simulink model "MISSILE_2angle"  (R2024b)
settings: Solver=ode4  StartTime=0.0  StopTime=100  FixedStep=0.01  RelTol=1e-3
values from neighbouring files (symbols this model uses):
  Ka = 4.5    [INITIAL_2angle.m]
  Kdc = 1.1    [INITIAL_2angle.m]
  Ki = 14.3    [INITIAL_2angle.m]
  Kr = -0.37    [INITIAL_2angle.m]
  L_M0 = 70*d2r    (= 1.2217304764)    [INITIAL_2angle.m]
  L_T0 = -2.5*d2r    (= -0.0436332312999)    [INITIAL_2angle.m]
  P_M0 = 50*d2r    (= 0.872664625997)    [INITIAL_2angle.m]
  P_T0 = 30*d2r    (= 0.523598775598)    [INITIAL_2angle.m]
  V_T = 600    [INITIAL_2angle.m]
  X_M0 = 0    [INITIAL_2angle.m]
  X_T0 = 0    [INITIAL_2angle.m]
  Y_T0 = 0    [INITIAL_2angle.m]
  Z_M0 = 0    [INITIAL_2angle.m]
  Z_T0 = 20000    [INITIAL_2angle.m]
libraries: simulink x1
settings Model: Creator=Administrator  LastModifiedBy=Administrator

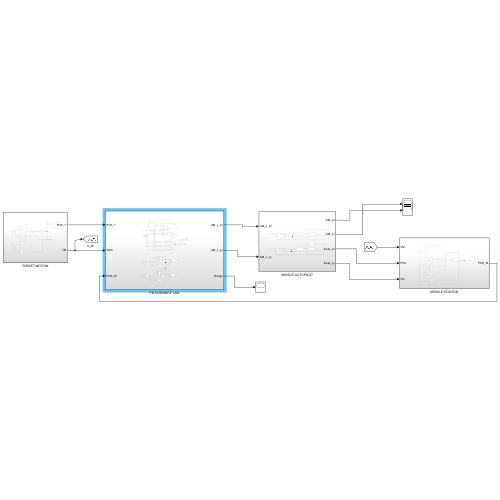
[thumbnail: Simulink's stored preview of the top-level diagram]
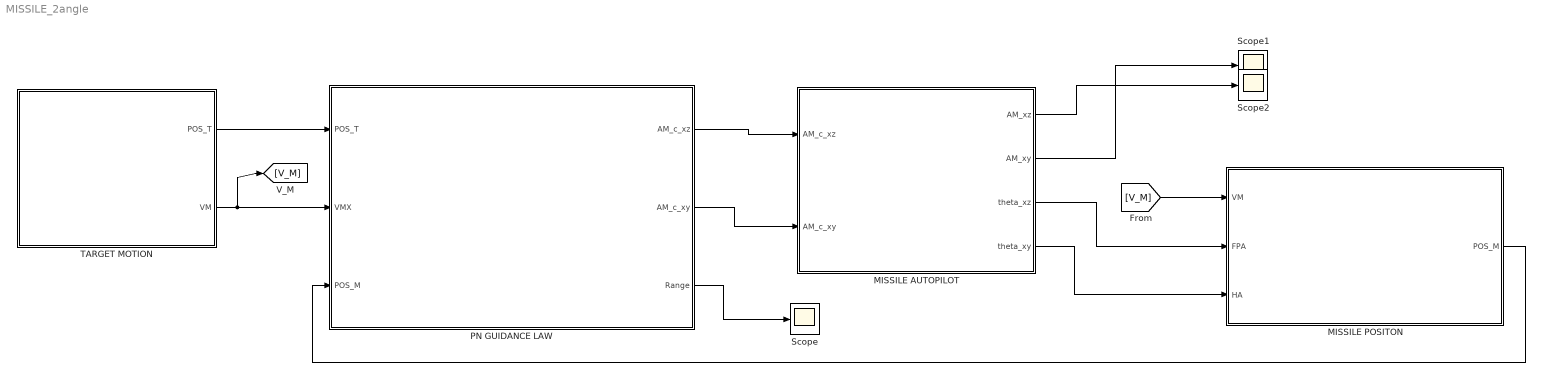
== system MISSILE_2angle ==
  MISSILE AUTOPILOT : Subsystem
  MISSILE POSITON : Subsystem
  PN GUIDANCE LAW : Subsystem
  Scope : Scope
  Scope1 : Scope
  Scope2 : Scope
  TARGET MOTION : Subsystem
  wires:
  TARGET MOTION/1(POS_T) -> PN GUIDANCE LAW/1(POS_T)
  TARGET MOTION/2(VM) -> [V_M], PN GUIDANCE LAW/2(VMX)
  [V_M] -> MISSILE POSITON/1(VM)
  MISSILE POSITON/1(POS_M) -> PN GUIDANCE LAW/3(POS_M)
  PN GUIDANCE LAW/1(AM_c_xz) -> MISSILE AUTOPILOT/1(AM_c_xz)
  MISSILE AUTOPILOT/1(AM_xz) -> Scope2/1
  MISSILE AUTOPILOT/3(theta_xz) -> MISSILE POSITON/2(FPA)
  PN GUIDANCE LAW/3(Range) -> Scope/1
  PN GUIDANCE LAW/2(AM_c_xy) -> MISSILE AUTOPILOT/2(AM_c_xy)
  MISSILE AUTOPILOT/2(AM_xy) -> Scope1/1
  MISSILE AUTOPILOT/4(theta_xy) -> MISSILE POSITON/3(HA)

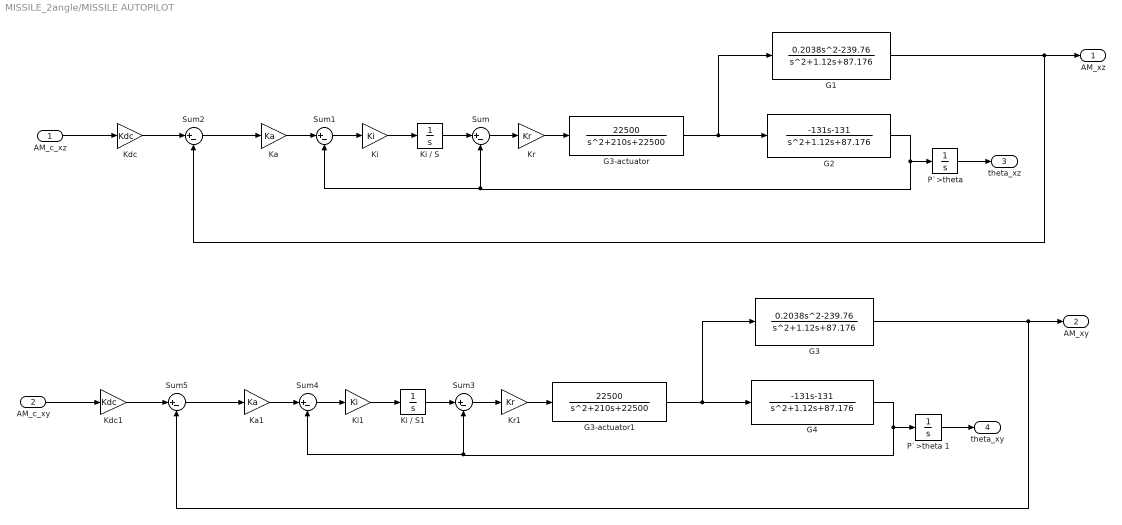
== system MISSILE_2angle/MISSILE AUTOPILOT ==
  AM_c_xz : Inport
  AM_c_xy : Inport  Port=2
  G1 : TransferFcn  Numerator=[0.2038 0 -239.76]  Denominator=[1 1.12 87.176]
  G2 : TransferFcn  Numerator=[-131 -131]  Denominator=[1 1.12 87.176]
  G3 : TransferFcn  Numerator=[0.2038 0 -239.76]  Denominator=[1 1.12 87.176]
  G3-actuator : TransferFcn  Numerator=[22500]  Denominator=[1 210 22500]
  G3-actuator1 : TransferFcn  Numerator=[22500]  Denominator=[1 210 22500]
  G4 : TransferFcn  Numerator=[-131 -131]  Denominator=[1 1.12 87.176]
  Ka : Gain  Gain=Ka
  Ka1 : Gain  Gain=Ka
  Kdc : Gain  Gain=Kdc
  Kdc1 : Gain  Gain=Kdc
  Ki : Gain  Gain=Ki
  Ki / S : Integrator
  Ki / S1 : Integrator
  Ki1 : Gain  Gain=Ki
  Kr : Gain  Gain=Kr
  Kr1 : Gain  Gain=Kr
  "P`>theta " : Integrator  InitialCondition=L_M0
  P`>theta 1 : Integrator  InitialCondition=P_M0
  Sum{,1..5} (6 alike) : Sum  Inputs=|+-
  AM_xz : Outport
  AM_xy : Outport  Port=2
  theta_xz : Outport  Port=3
  theta_xy : Outport  Port=4
  wires:
  Ki / S/1 -> Sum/1
  G1/1 -> AM_xz/1, Sum2/2
  Kr/1 -> G3-actuator/1
  "P`>theta "/1 -> theta_xz/1
  Ka/1 -> Sum1/1
  G3-actuator/1 -> G1/1, G2/1
  Sum1/1 -> Ki/1
  G2/1 -> "P`>theta "/1, Sum1/2, Sum/2
  Kdc/1 -> Sum2/1
  Ki/1 -> Ki / S/1
  Sum/1 -> Kr/1
  Sum2/1 -> Ka/1
  AM_c_xz/1 -> Kdc/1
  P`>theta 1/1 -> theta_xy/1
  Sum3/1 -> Kr1/1
  G4/1 -> P`>theta 1/1, Sum4/2, Sum3/2
  G3-actuator1/1 -> G3/1, G4/1
  AM_c_xy/1 -> Kdc1/1
  Kr1/1 -> G3-actuator1/1
  Ki1/1 -> Ki / S1/1
  G3/1 -> AM_xy/1, Sum5/2
  Ka1/1 -> Sum4/1
  Kdc1/1 -> Sum5/1
  Ki / S1/1 -> Sum3/1
  Sum4/1 -> Ki1/1
  Sum5/1 -> Ka1/1

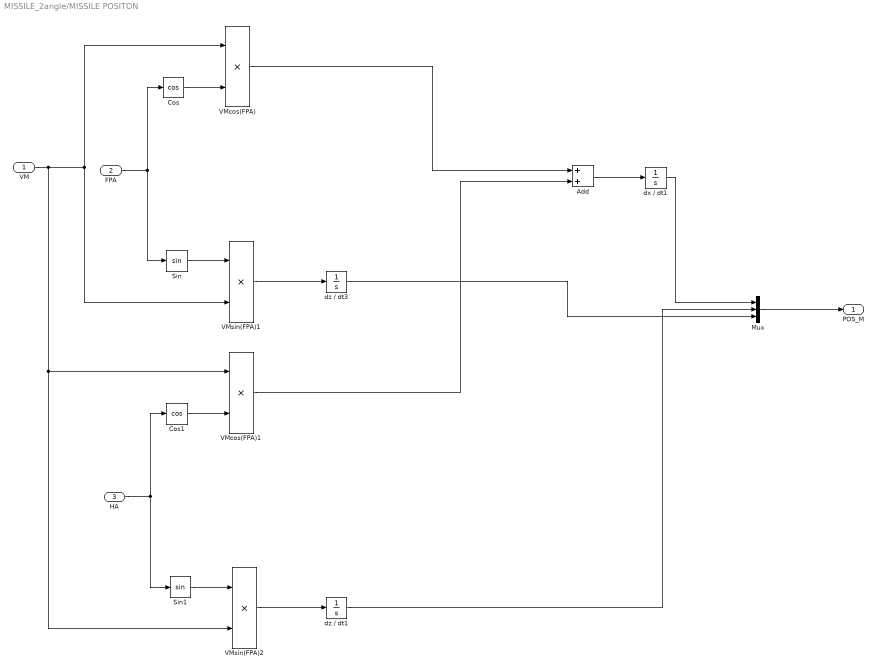
== system MISSILE_2angle/MISSILE POSITON ==
  VM : Inport
  FPA : Inport  Port=2
  HA : Inport  Port=3
  Add : Sum
  Cos : Trigonometry  Operator=cos
  Cos1 : Trigonometry  Operator=cos
  Mux : Mux  Inputs=3
  Sin : Trigonometry
  Sin1 : Trigonometry
  VMcos(FPA) : Product
  VMcos(FPA)1 : Product
  VMsin(FPA)1 : Product
  VMsin(FPA)2 : Product
  dx / dt1 : Integrator  InitialCondition=X_M0
  dz / dt1 : Integrator  InitialCondition=Z_M0
  dz / dt3 : Integrator  InitialCondition=Z_M0
  POS_M : Outport
  wires:
  Sin/1 -> VMsin(FPA)1/1
  Mux/1 -> POS_M/1
  Cos/1 -> VMcos(FPA)/2
  VM/1 -> VMsin(FPA)2/2, VMcos(FPA)1/1, VMsin(FPA)1/2, VMcos(FPA)/1
  FPA/1 -> Sin/1, Cos/1
  Sin1/1 -> VMsin(FPA)2/1
  Cos1/1 -> VMcos(FPA)1/2
  HA/1 -> Sin1/1, Cos1/1
  VMsin(FPA)1/1 -> dz / dt3/1
  VMsin(FPA)2/1 -> dz / dt1/1
  VMcos(FPA)/1 -> Add/1
  Add/1 -> dx / dt1/1
  VMcos(FPA)1/1 -> Add/2
  dz / dt3/1 -> Mux/3
  dz / dt1/1 -> Mux/2
  dx / dt1/1 -> Mux/1

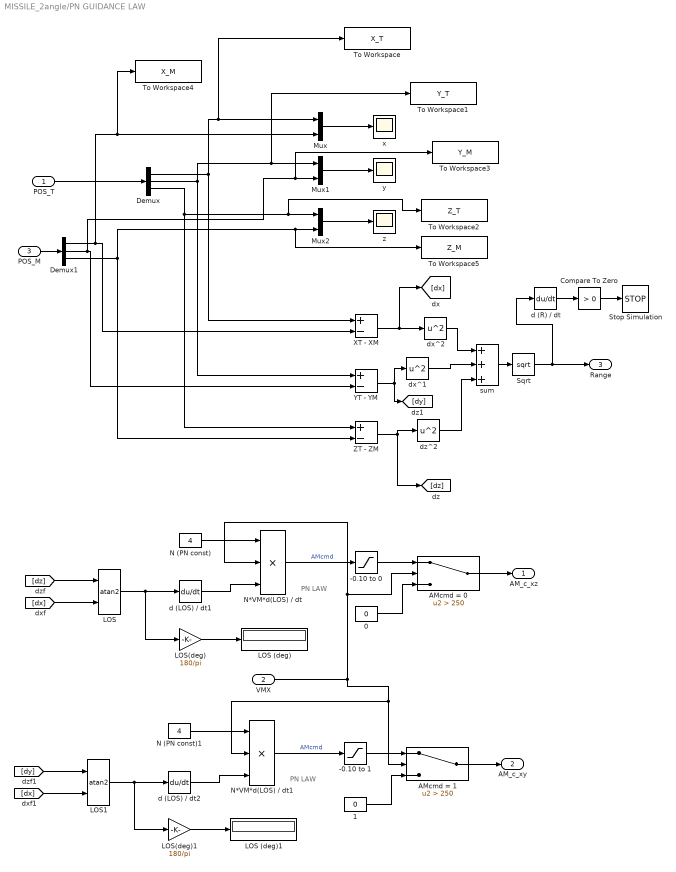
== system MISSILE_2angle/PN GUIDANCE LAW ==
  note: PN LAW
  note: PN LAW
  POS_T : Inport
  VMX : Inport  Port=2
  POS_M : Inport  Port=3
  -0.10 to 0 : Saturate  UpperLimit=1  LowerLimit=-0.1
  -0.10 to 1 : Saturate  UpperLimit=1
  0 : Constant  Value=0
  1 : Constant  Value=0
  AMcmd = 0 : Switch  Criteria=u2 > Threshold  Threshold=250  SaturateOnIntegerOverflow=off  InputSameDT=off
  AMcmd = 1 : Switch  Criteria=u2 > Threshold  Threshold=250  SaturateOnIntegerOverflow=off  InputSameDT=off
  Compare To Zero : simulink/Logic and Bit Operations/Compare To Zero  relop=>  OutDataTypeStr=boolean
  Demux : Demux  Outputs=3
  Demux1 : Demux  Outputs=3
  LOS : Trigonometry  Operator=atan2
  LOS (deg) : Display
  LOS (deg)1 : Display
  LOS(deg) : Gain  Gain=180/pi
  LOS(deg)1 : Gain  Gain=180/pi
  LOS1 : Trigonometry  Operator=atan2
  Mux : Mux  Inputs=2
  Mux1 : Mux  Inputs=2
  Mux2 : Mux  Inputs=2
  N (PN const) : Constant  Value=4
  N (PN const)1 : Constant  Value=4
  N*VM*d(LOS) / dt : Product  Inputs=3
  N*VM*d(LOS) / dt1 : Product  Inputs=3
  Sqrt : Sqrt
  Stop Simulation : Stop
  To Workspace : ToWorkspace  VariableName=X_T  SaveFormat=Timeseries  SampleTime=-1
  To Workspace1 : ToWorkspace  VariableName=Y_T  SaveFormat=Timeseries  SampleTime=-1
  To Workspace2 : ToWorkspace  VariableName=Z_T  SaveFormat=Timeseries  SampleTime=-1
  To Workspace3 : ToWorkspace  VariableName=Y_M  SaveFormat=Timeseries  SampleTime=-1
  To Workspace4 : ToWorkspace  VariableName=X_M  SaveFormat=Timeseries  SampleTime=-1
  To Workspace5 : ToWorkspace  VariableName=Z_M  SaveFormat=Timeseries  SampleTime=-1
  XT - XM : Sum  Inputs=+-
  YT - YM : Sum  Inputs=+-
  ZT - ZM : Sum  Inputs=+-
  d (LOS) / dt1 : Derivative
  d (LOS) / dt2 : Derivative
  d (R) / dt : Derivative
  dx^1 : Math  Operator=square
  dx^2 : Math  Operator=square
  dz^2 : Math  Operator=square
  sum : Sum  Inputs=+++
  x : Scope
  y : Scope
  z : Scope
  AM_c_xz : Outport
  AM_c_xy : Outport  Port=2
  Range : Outport  Port=3
  wires:
  POS_T/1 -> Demux/1
  d (R) / dt/1 -> Compare To Zero/1
  0/1 -> AMcmd = 0/3
  ZT - ZM/1 -> [dz], dz^2/1
  N*VM*d(LOS) / dt/1 -> -0.10 to 0/1  "AMcmd"
  -0.10 to 0/1 -> AMcmd = 0/1
  XT - XM/1 -> [dx], dx^2/1
  LOS/1 -> LOS(deg)/1, d (LOS) / dt1/1
  AMcmd = 0/1 -> AM_c_xz/1
  N (PN const)/1 -> N*VM*d(LOS) / dt/1
  [dx] -> LOS/2
  d (LOS) / dt1/1 -> N*VM*d(LOS) / dt/3
  dx^2/1 -> sum/1
  Compare To Zero/1 -> Stop Simulation/1
  [dz] -> LOS/1
  POS_M/1 -> Demux1/1
  LOS(deg)/1 -> LOS (deg)/1
  Mux1/1 -> y/1
  Mux/1 -> x/1
  dz^2/1 -> sum/3
  Demux/1 -> XT - XM/1, To Workspace/1, Mux/1
  Demux/2 -> To Workspace1/1, Mux1/1, YT - YM/1
  Demux/3 -> To Workspace2/1, Mux2/1, ZT - ZM/1
  Demux1/1 -> Mux/2, To Workspace4/1, XT - XM/2
  Demux1/2 -> To Workspace3/1, Mux1/2, YT - YM/2
  Demux1/3 -> ZT - ZM/2, To Workspace5/1, Mux2/2
  Mux2/1 -> z/1
  YT - YM/1 -> [dy], dx^1/1
  dx^1/1 -> sum/2
  AMcmd = 1/1 -> AM_c_xy/1
  LOS(deg)1/1 -> LOS (deg)1/1
  -0.10 to 1/1 -> AMcmd = 1/1
  N (PN const)1/1 -> N*VM*d(LOS) / dt1/1
  1/1 -> AMcmd = 1/3
  LOS1/1 -> LOS(deg)1/1, d (LOS) / dt2/1
  [dy] -> LOS1/1
  d (LOS) / dt2/1 -> N*VM*d(LOS) / dt1/3
  [dx] -> LOS1/2
  N*VM*d(LOS) / dt1/1 -> -0.10 to 1/1  "AMcmd"
  VMX/1 -> N*VM*d(LOS) / dt/2, AMcmd = 0/2, N*VM*d(LOS) / dt1/2, AMcmd = 1/2
  sum/1 -> Sqrt/1
  Sqrt/1 -> Range/1, d (R) / dt/1

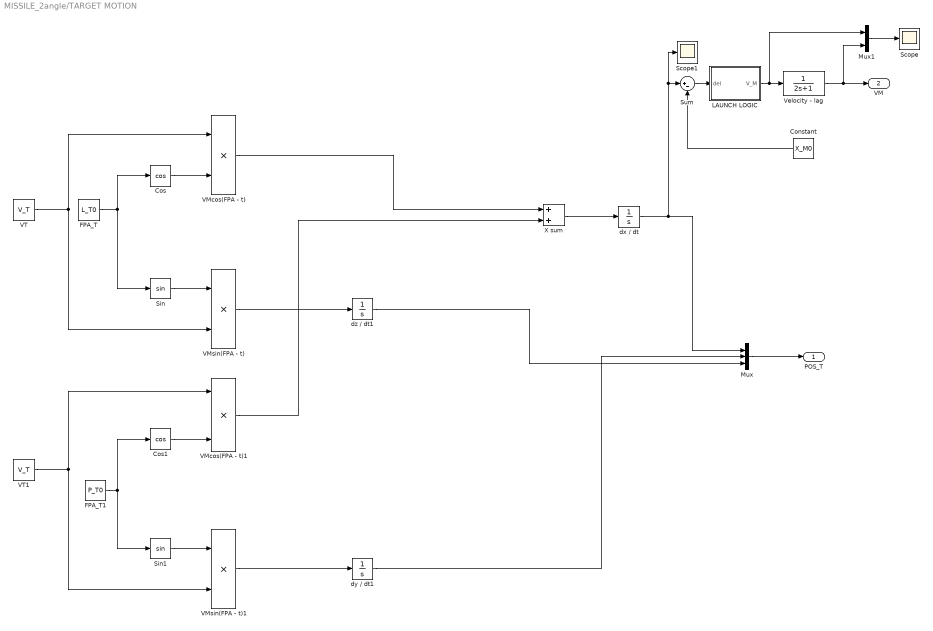
== system MISSILE_2angle/TARGET MOTION ==
  Constant : Constant  Value=X_M0
  Cos : Trigonometry  Operator=cos
  Cos1 : Trigonometry  Operator=cos
  FPA_T : Constant  Value=L_T0
  FPA_T1 : Constant  Value=P_T0
  LAUNCH LOGIC : MATLAB Function  TreatAsAtomicUnit=on
  Mux : Mux  Inputs=3
  Mux1 : Mux  Inputs=2
  Scope : Scope
  Scope1 : Scope
  Sin : Trigonometry
  Sin1 : Trigonometry
  Sum : Sum  Inputs=|+-
  VMcos(FPA - t) : Product
  VMcos(FPA - t)1 : Product  Inputs=3
  VMsin(FPA - t) : Product
  VMsin(FPA - t)1 : Product
  VT : Constant  Value=V_T
  VT1 : Constant  Value=V_T
  "Velocity - lag " : TransferFcn  Denominator=[2 1]
  X sum : Sum
  dx / dt : Integrator  InitialCondition=X_T0
  dy / dt1 : Integrator  InitialCondition=Y_T0
  dz / dt1 : Integrator  InitialCondition=Z_T0
  POS_T : Outport
  VM : Outport  Port=2
  wires:
  FPA_T/1 -> Sin/1, Cos/1
  VT/1 -> VMsin(FPA - t)/2, VMcos(FPA - t)/1
  Sum/1 -> LAUNCH LOGIC/1(del)
  Mux1/1 -> Scope/1
  LAUNCH LOGIC/1(V_M) -> Mux1/1, "Velocity - lag "/1
  Cos/1 -> VMcos(FPA - t)/2
  Sin/1 -> VMsin(FPA - t)/1
  "Velocity - lag "/1 -> VM/1, Mux1/2
  Mux/1 -> POS_T/1
  VT1/1 -> VMsin(FPA - t)1/2, VMcos(FPA - t)1/1
  FPA_T1/1 -> Cos1/1, Sin1/1
  Cos1/1 -> VMcos(FPA - t)1/3
  Sin1/1 -> VMsin(FPA - t)1/1
  VMsin(FPA - t)/1 -> dz / dt1/1
  VMsin(FPA - t)1/1 -> dy / dt1/1
  VMcos(FPA - t)/1 -> X sum/1
  VMcos(FPA - t)1/1 -> X sum/2
  Constant/1 -> Sum/2
  dy / dt1/1 -> Mux/2
  dz / dt1/1 -> Mux/3
  X sum/1 -> dx / dt/1
  dx / dt/1 -> Scope1/1, Sum/1, Mux/1

== matlab function MISSILE_2angle/TARGET MOTION/LAUNCH LOGIC ==
  settings: updateMethod=DISCRETE
  data: del input; V_M output
function V_M = fcn(del)

persistent f
persistent Vel

if isempty(f)
    f = 0;
end
if isempty(Vel)
    Vel = 0;
end

if f ==0 && del > -200
    f = 1;
    Vel = 1000; %missile speed
end


V_M = Vel;
